simulink model "KCC_Model"  (R2023b)
settings: Solver=VariableStepAuto  StartTime=0.0  StopTime=10.0  RelTol=1e-3
libraries: dspxfrm3 x3
settings Model: Creator=samkramer  LastModifiedBy=samkramer

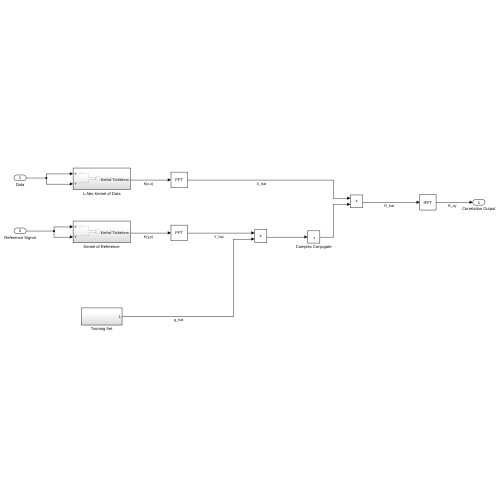
[thumbnail: Simulink's stored preview of the top-level diagram]
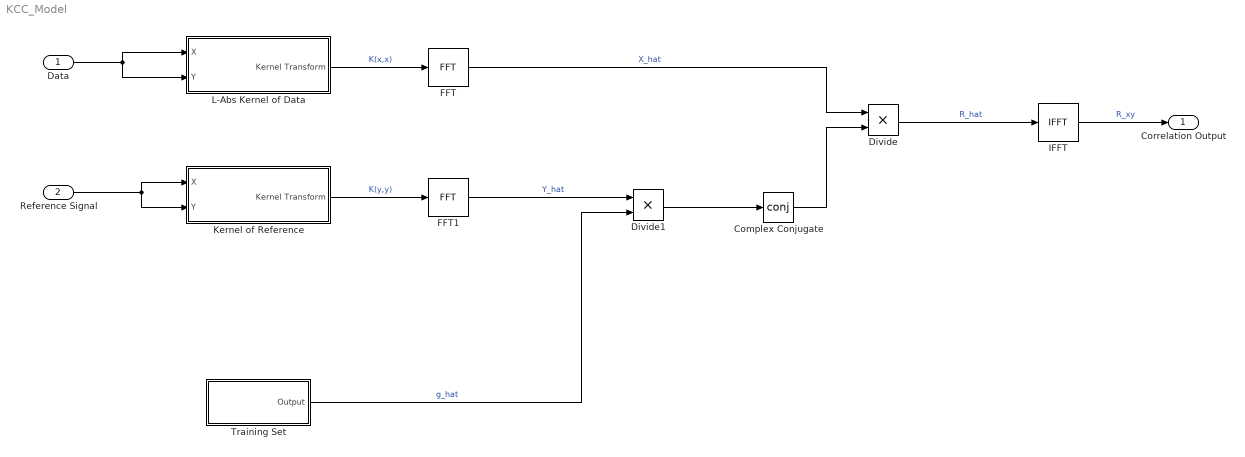
== system KCC_Model ==
  Data : Inport
  Reference Signal : Inport  Port=2
  Complex Conjugate : Math  Operator=conj
  Divide : Product  Inputs=**
  Divide1 : Product  Inputs=**
  FFT : dspxfrm3/FFT  FFTImplementation=Auto  CompMethod=Table lookup  TableOpt=NEW  TableOptActive=Speed  BitRevOrder=off  Normalize=off  InheritFFTLength=on  FFTLength=64  WrapInput=on  roundingMode=Floor  overflowMode=off  firstCoeffDataTypeStr=Inherit: Same word length as input  firstCoeffLastDataTypeStr=Inherit: Same word length as input  outputMin=[]  outputMax=[]
  FFT1 : dspxfrm3/FFT  FFTImplementation=Auto  CompMethod=Table lookup  TableOpt=NEW  TableOptActive=Speed  BitRevOrder=off  Normalize=off  InheritFFTLength=on  FFTLength=64  WrapInput=on  roundingMode=Floor  overflowMode=off  firstCoeffDataTypeStr=Inherit: Same word length as input  firstCoeffLastDataTypeStr=Inherit: Same word length as input  outputMin=[]  outputMax=[]
  IFFT : dspxfrm3/IFFT  FFTImplementation=Auto  CompMethod=Table lookup  TableOpt=NEW  TableOptActive=Speed  BitRevOrder=off  cs_in=off  Normalize=on  InheritFFTLength=on  FFTLength=64  WrapInput=on  mode=Complex  outSamplingMode=Sample based  roundingMode=Floor  overflowMode=off  firstCoeffDataTypeStr=Inherit: Same word length as input  firstCoeffLastDataTypeStr=Inherit: Same word length as input  outputMin=[]  outputMax=[]
  Kernel of Reference : Subsystem
  L-Abs Kernel of Data : Subsystem
  Training Set : Subsystem
  Correlation Output : Outport
  wires:
  Data/1 -> L-Abs Kernel of Data/1(X), L-Abs Kernel of Data/2(Y)
  Reference Signal/1 -> Kernel of Reference/2(Y), Kernel of Reference/1(X)
  L-Abs Kernel of Data/1(Kernel Transform) -> FFT/1  "K(x,x)"
  FFT/1 -> Divide/1  "X_hat"
  Kernel of Reference/1(Kernel Transform) -> FFT1/1  "K(y,y)"
  FFT1/1 -> Divide1/1  "Y_hat"
  Complex Conjugate/1 -> Divide/2
  Training Set/1(Output) -> Divide1/2  "g_hat"
  Divide1/1 -> Complex Conjugate/1
  Divide/1 -> IFFT/1  "R_hat"
  IFFT/1 -> Correlation Output/1  "R_xy"

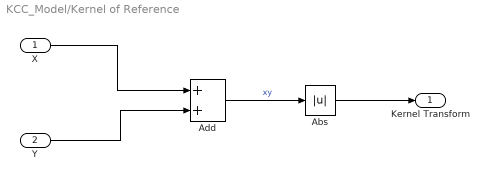
== system KCC_Model/Kernel of Reference ==
  X : Inport
  Y : Inport  Port=2
  Abs : Abs  SaturateOnIntegerOverflow=off
  Add : Sum
  Kernel Transform : Outport
  wires:
  X/1 -> Add/1
  Add/1 -> Abs/1  "xy"
  Abs/1 -> Kernel Transform/1
  Y/1 -> Add/2

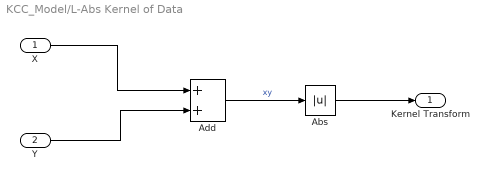
== system KCC_Model/L-Abs Kernel of Data ==
  X : Inport
  Y : Inport  Port=2
  Abs : Abs  SaturateOnIntegerOverflow=off
  Add : Sum
  Kernel Transform : Outport
  wires:
  X/1 -> Add/1
  Add/1 -> Abs/1  "xy"
  Abs/1 -> Kernel Transform/1
  Y/1 -> Add/2

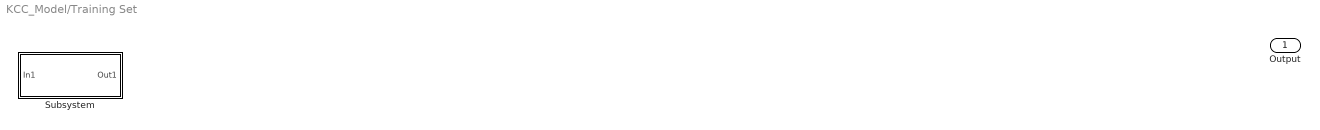
== system KCC_Model/Training Set ==
  Subsystem : Subsystem
  Output : Outport

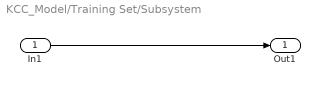
== system KCC_Model/Training Set/Subsystem ==
  In1 : Inport
  Out1 : Outport
  wires:
  In1/1 -> Out1/1
